simulink subsystem "Correct"  (R2023a)
settings: Solver=VariableStepAuto  StartTime=0.0  StopTime=10.0  RelTol=1e-3
values from neighbouring files (symbols this model uses):
  ak0 = 1    [main.m]
  ak1 = 0.5    [main.m]
  ap0 = 1    [main.m]
  ap1 = 0.001    [main.m]
  bk0 = 0    [main.m]
  bk1 = 0.5    [main.m]
  bp0 = 1    [main.m]
  bp1 = 0.001    [main.m]
  Kc = 0.0015    [main.m]
  Ki = 0.0003    [main.m]
  Kk = 22500    [main.m]
settings Model: Creator=ycheb  LastModifiedBy=ycheb

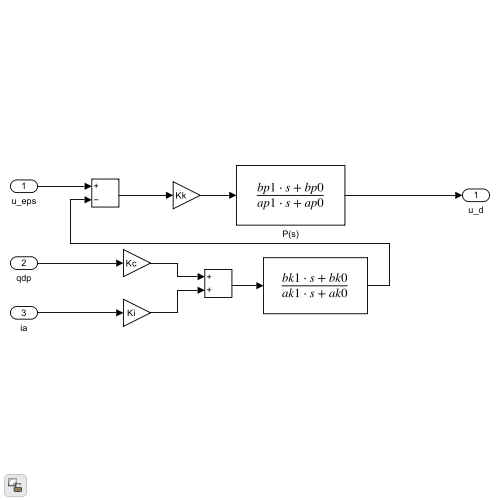
[thumbnail: Simulink's stored preview of the top-level diagram]
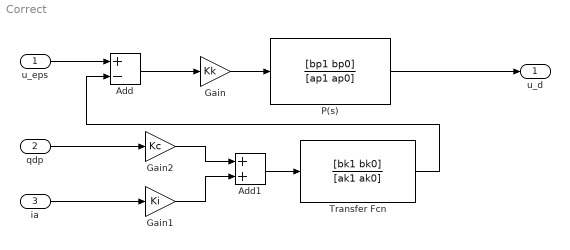
== system Correct ==
  u_eps : Inport
  qdp : Inport  Port=2
  ia : Inport  Port=3
  Add : Sum  Inputs=+-
  Add1 : Sum
  Gain : Gain  Gain=Kk
  Gain1 : Gain  Gain=Ki
  Gain2 : Gain  Gain=Kc
  P(s) : TransferFcn  Numerator=[bp1 bp0]  Denominator=[ap1 ap0]
  Transfer Fcn : TransferFcn  Numerator=[bk1 bk0]  Denominator=[ak1 ak0]
  u_d : Outport
  wires:
  u_eps/1 -> Add/1
  Add/1 -> Gain/1
  Gain/1 -> P(s)/1
  P(s)/1 -> u_d/1
  ia/1 -> Gain1/1
  qdp/1 -> Gain2/1
  Gain2/1 -> Add1/1
  Gain1/1 -> Add1/2
  Add1/1 -> Transfer Fcn/1
  Transfer Fcn/1 -> Add/2
